simulink model "cdip_lqr_servo_sim"  (R2013a)
settings: Solver=ode1  StartTime=0.0  StopTime=t_end  FixedStep=0.001  RelTol=1e-3
values from neighbouring files (symbols this model uses):
  ac = 6.25    [p1c62_ex1_cart_p_step.m]    (also in p1c62_ex2_cart_pi_ramp.m; p1c62_ex3_cart_p_step_dis.m; p1c62_ex4_cart_pi_step_dis.m)
  bc = 4.36    [p1c62_ex1_cart_p_step.m]    (also in p1c62_ex2_cart_pi_ramp.m; p1c62_ex3_cart_p_step_dis.m; p1c62_ex4_cart_pi_step_dis.m)
  d0 = 3    [p1c62_ex3_cart_p_step_dis.m]    (also in p1c62_ex4_cart_pi_step_dis.m; p1c63_ex5_cdip_lqr_servo.m = 5)
  dtheta_0 = 0    [p1c63_ex5_cdip_lqr_servo.m]
  dz_0 = 0    [p1c63_ex5_cdip_lqr_servo.m]
  K1 = Kt(1:4)    [p1c63_ex5_cdip_lqr_servo.m]
  K2 = Kt(5)    [p1c63_ex5_cdip_lqr_servo.m]
  r0 = 0.5    [p1c62_ex1_cart_p_step.m]    (also in p1c62_ex2_cart_pi_ramp.m = 0.1; p1c62_ex3_cart_p_step_dis.m; p1c62_ex4_cart_pi_step_dis.m; p1c63_ex5_cdip_lqr_servo.m)
  t_dis = 2.5    [p1c62_ex3_cart_p_step_dis.m]    (also in p1c62_ex4_cart_pi_step_dis.m; p1c63_ex5_cdip_lqr_servo.m)
  theta_0 = 0    [p1c63_ex5_cdip_lqr_servo.m]
  z_0 = 0    [p1c63_ex5_cdip_lqr_servo.m]
undefined symbols (not defined in the file or in its folder): g, Jp, lp, mp, mup
settings Model: Creator=kawata  LastModifiedBy=kawata
settings DataIOCC: LimitDataPoints=off  SignalLoggingSaveFormat=ModelDataLogs
settings OptimizationCC: ExpressionDepthLimit=2147483647
settings DebuggingCC: FcnCallInpInsideContextMsg=UseLocalSettings
settings GRTTargetCC: CombineOutputUpdateFcns=off  GRTInterface=on

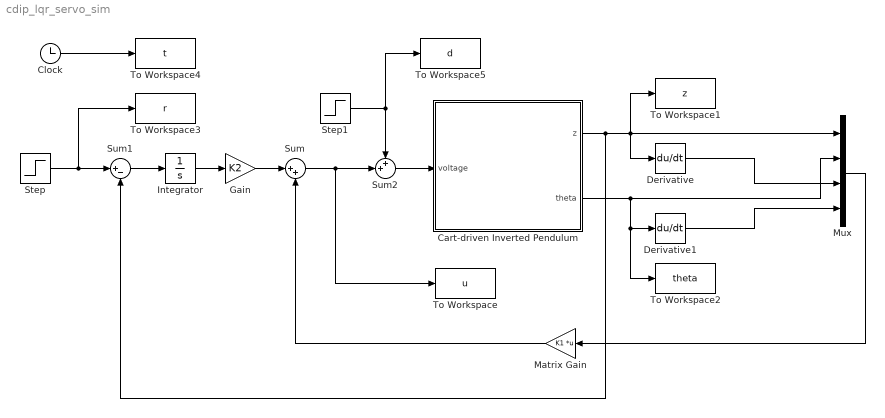
== system cdip_lqr_servo_sim ==
  Cart-driven Inverted Pendulum : Subsystem
      mask Display: image(imread('cdip.jpg'),'center')
  Clock : Clock
  Derivative : Derivative
  Derivative1 : Derivative
  Gain : Gain  Gain=K2  SaturateOnIntegerOverflow=on  OutDataTypeStr=Inherit: Same as input  ParamDataTypeStr=Inherit: Same as input
  Integrator : Integrator
  Matrix Gain : Gain  Gain=K1  Multiplication=Matrix(K*u)  SaturateOnIntegerOverflow=on  OutDataTypeStr=Inherit: Same as input  ParamDataTypeStr=Inherit: Same as input
  Mux : Mux
  Step : Step  Time=0  After=r0  SampleTime=0
  Step1 : Step  Time=t_dis  After=d0  SampleTime=0
  Sum : Sum  Inputs=|++  SaturateOnIntegerOverflow=on  InputSameDT=on  OutDataTypeStr=Inherit: Same as first input
  Sum1 : Sum  Inputs=|+-  SaturateOnIntegerOverflow=on  InputSameDT=on  OutDataTypeStr=Inherit: Same as first input
  Sum2 : Sum  Inputs=++|  SaturateOnIntegerOverflow=on  InputSameDT=on  OutDataTypeStr=Inherit: Same as first input
  To Workspace : ToWorkspace  VariableName=u  SampleTime=-1
  To Workspace1 : ToWorkspace  VariableName=z  SampleTime=-1
  To Workspace2 : ToWorkspace  VariableName=theta  SampleTime=-1
  To Workspace3 : ToWorkspace  VariableName=r  SampleTime=-1
  To Workspace4 : ToWorkspace  VariableName=t  SampleTime=-1
  To Workspace5 : ToWorkspace  VariableName=d  SampleTime=-1
  wires:
  Mux/1 -> Matrix Gain/1
  Matrix Gain/1 -> Sum/2
  Sum1/1 -> Integrator/1
  Integrator/1 -> Gain/1
  Gain/1 -> Sum/1
  Sum/1 -> Sum2/2, To Workspace/1
  Step/1 -> Sum1/1, To Workspace3/1
  Step1/1 -> To Workspace5/1, Sum2/1
  Sum2/1 -> Cart-driven Inverted Pendulum/1(voltage)
  Clock/1 -> To Workspace4/1
  Cart-driven Inverted Pendulum/1(z) -> To Workspace1/1, Derivative/1, Mux/1, Sum1/2
  Cart-driven Inverted Pendulum/2(theta) -> To Workspace2/1, Derivative1/1, Mux/2
  Derivative/1 -> Mux/3
  Derivative1/1 -> Mux/4

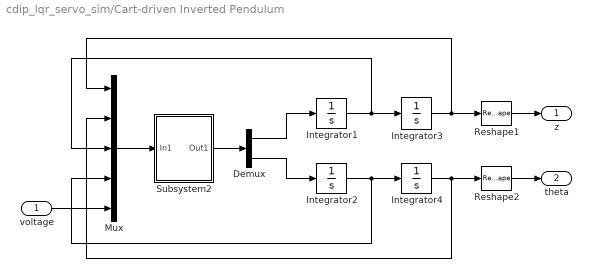
== system cdip_lqr_servo_sim/Cart-driven Inverted Pendulum ==
  voltage : Inport
  Demux : Demux  Outputs=2
  Integrator1 : Integrator  InitialCondition=dz_0
  Integrator2 : Integrator  InitialCondition=dtheta_0
  Integrator3 : Integrator  InitialCondition=z_0
  Integrator4 : Integrator  InitialCondition=theta_0
  Mux : Mux  Inputs=5
  Reshape1 : Reshape
  Reshape2 : Reshape
  Subsystem2 : Subsystem
  z : Outport
  theta : Outport  Port=2
  wires:
  Reshape2/1 -> theta/1
  Reshape1/1 -> z/1
  voltage/1 -> Mux/5
  Integrator4/1 -> Mux/2, Reshape2/1
  Integrator3/1 -> Mux/1, Reshape1/1
  Integrator2/1 -> Integrator4/1, Mux/4
  Integrator1/1 -> Integrator3/1, Mux/3
  Demux/2 -> Integrator2/1
  Demux/1 -> Integrator1/1
  Mux/1 -> Subsystem2/1(In1)
  Subsystem2/1(Out1) -> Demux/1

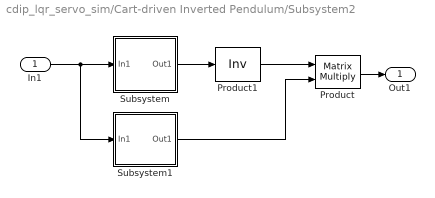
== system cdip_lqr_servo_sim/Cart-driven Inverted Pendulum/Subsystem2 ==
  In1 : Inport
  Product : Product  Multiplication=Matrix(*)  SaturateOnIntegerOverflow=on  InputSameDT=on  OutDataTypeStr=Inherit: Same as first input
  Product1 : Product  Inputs=/  Multiplication=Matrix(*)  SaturateOnIntegerOverflow=on  InputSameDT=on  OutDataTypeStr=Inherit: Same as first input
  Subsystem : Subsystem
  Subsystem1 : Subsystem
  Out1 : Outport
  wires:
  Subsystem/1(Out1) -> Product1/1
  Product1/1 -> Product/1
  Subsystem1/1(Out1) -> Product/2
  In1/1 -> Subsystem/1(In1), Subsystem1/1(In1)
  Product/1 -> Out1/1

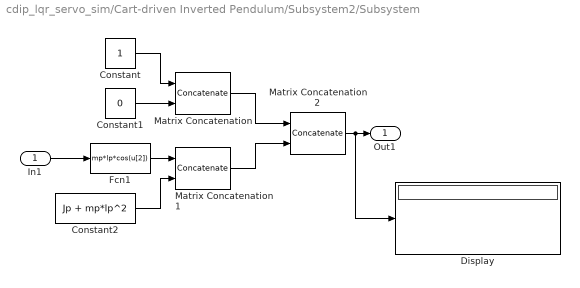
== system cdip_lqr_servo_sim/Cart-driven Inverted Pendulum/Subsystem2/Subsystem ==
  In1 : Inport
  Constant : Constant
  Constant1 : Constant  Value=0
  Constant2 : Constant  Value=Jp + mp*lp^2
  Display : Display
  Fcn1 : Fcn  Expr=mp*lp*cos(u[2])
  Matrix Concatenation : Concatenate  Mode=Multidimensional array  ConcatenateDimension=2
  Matrix Concatenation1 : Concatenate  Mode=Multidimensional array  ConcatenateDimension=2
  Matrix Concatenation2 : Concatenate  Mode=Multidimensional array
  Out1 : Outport
  wires:
  Constant2/1 -> Matrix Concatenation1/2
  Fcn1/1 -> Matrix Concatenation1/1
  In1/1 -> Fcn1/1
  Matrix Concatenation/1 -> Matrix Concatenation2/1
  Matrix Concatenation1/1 -> Matrix Concatenation2/2
  Matrix Concatenation2/1 -> Display/1, Out1/1
  Constant/1 -> Matrix Concatenation/1
  Constant1/1 -> Matrix Concatenation/2

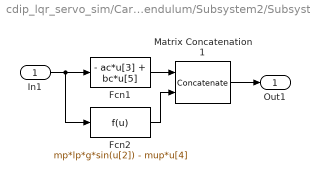
== system cdip_lqr_servo_sim/Cart-driven Inverted Pendulum/Subsystem2/Subsystem1 ==
  In1 : Inport
  Fcn1 : Fcn  Expr=- ac*u[3] + bc*u[5]
  Fcn2 : Fcn  Expr=mp*lp*g*sin(u[2]) - mup*u[4]
  Matrix Concatenation1 : Concatenate  Mode=Multidimensional array
  Out1 : Outport
  wires:
  Fcn2/1 -> Matrix Concatenation1/2
  Fcn1/1 -> Matrix Concatenation1/1
  In1/1 -> Fcn2/1, Fcn1/1
  Matrix Concatenation1/1 -> Out1/1
